simulink model "motor_modeli"  (R2024a)
settings: Solver=ode23  StartTime=0.0  StopTime=100  FixedStep=0.5  RelTol=1e-3
values from neighbouring files (symbols this model uses):
  B = 0.0001    [Motor_verileri.m]    (also in deneme1_proje_z.m)
  J = 0.004    [Motor_verileri.m]    (also in deneme1_proje_z.m = 0.0001)
  Kd = 0.000033    (= 3.3e-05)    [Motor_verileri.m]
  Ke = 0.12    [Motor_verileri.m]    (also in deneme1_proje_z.m = 0.05)
  Ki = 2.43    [Motor_verileri.m]
  Kp = 0.0114    [Motor_verileri.m]
  Kt = 0.12    [Motor_verileri.m]    (also in deneme1_proje_z.m = 0.05)
  L = 0.00005    (= 5e-05)    [Motor_verileri.m]    (also in deneme1_proje_z.m)
  R = 0.017    [Motor_verileri.m]    (also in deneme1_proje_z.m)
libraries: simulink x1
settings Model: Creator=user  LastModifiedBy=user

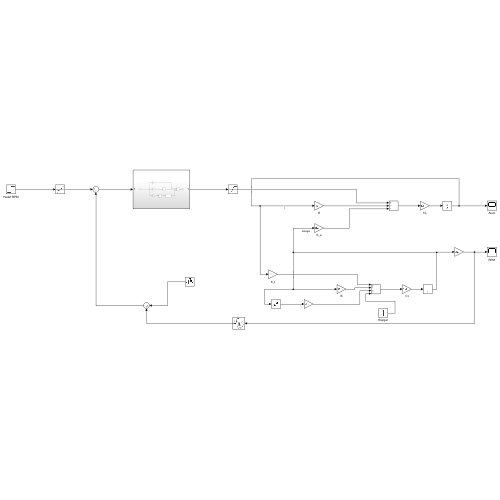
[thumbnail: Simulink's stored preview of the top-level diagram]
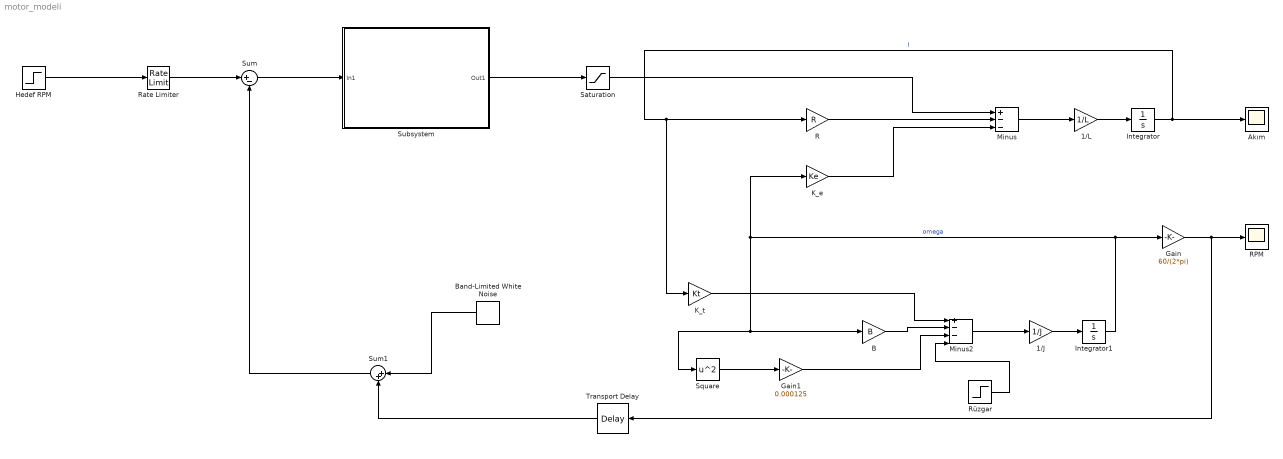
== system motor_modeli ==
  1/J : Gain  Gain=1/J
  1/L : Gain  Gain=1/L
  Akım : Scope
  B : Gain  Gain=B
  Band-Limited White Noise : simulink/Sources/Band-Limited White Noise  Cov=[0.0001]  Ts=0.1  seed=[23341]
  Gain : Gain  Gain=60/(2*pi)
  Gain1 : Gain  Gain=0.000125
  Hedef RPM : Step  Time=0.1  After=3000  SampleTime=0
  Integrator : Integrator
  Integrator1 : Integrator
  K_e : Gain  Gain=Ke
  K_t : Gain  Gain=Kt
  Minus : Sum  Inputs=+--
  Minus2 : Sum  Inputs=+---
  R : Gain  Gain=R
  RPM : Scope
  Rate Limiter : RateLimiter  RisingSlewLimit=1000  FallingSlewLimit=-1000  SampleTimeMode=inherited
  Rüzgar : Step  Time=0.5  After=5  SampleTime=0
  Saturation : Saturate  UpperLimit=60  LowerLimit=0
  Square : Math  Operator=square
  Subsystem : Subsystem
  Sum : Sum  Inputs=|+-
  Sum1 : Sum  Inputs=|++
  Transport Delay : TransportDelay  DelayTime=0.005
  wires:
  R/1 -> Minus/2
  K_e/1 -> Minus/3
  Minus/1 -> 1/L/1
  1/L/1 -> Integrator/1
  Integrator/1 -> K_t/1, R/1, Akım/1  "I"
  K_t/1 -> Minus2/1
  Minus2/1 -> 1/J/1
  Gain1/1 -> Minus2/3
  Integrator1/1 -> K_e/1, Square/1, B/1, Gain/1  "omega"
  B/1 -> Minus2/2
  1/J/1 -> Integrator1/1
  Square/1 -> Gain1/1
  Hedef RPM/1 -> Rate Limiter/1
  Sum/1 -> Subsystem/1(In1)
  Subsystem/1(Out1) -> Saturation/1
  Saturation/1 -> Minus/1
  Band-Limited White Noise/1 -> Sum1/1
  Gain/1 -> Transport Delay/1, RPM/1
  Rüzgar/1 -> Minus2/4
  Transport Delay/1 -> Sum1/2
  Rate Limiter/1 -> Sum/1
  Sum1/1 -> Sum/2

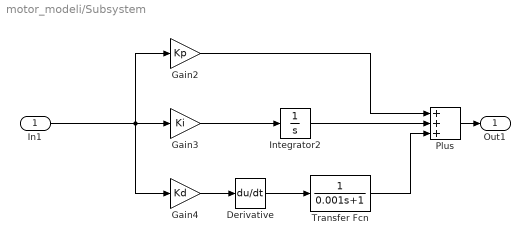
== system motor_modeli/Subsystem ==
  In1 : Inport
  Derivative : Derivative
  Gain2 : Gain  Gain=Kp
  Gain3 : Gain  Gain=Ki
  Gain4 : Gain  Gain=Kd
  Integrator2 : Integrator  LimitOutput=on  UpperSaturationLimit=60  LowerSaturationLimit=0
  Plus : Sum  Inputs=+++
  Transfer Fcn : TransferFcn  Denominator=[0.001 1]
  Out1 : Outport
  wires:
  In1/1 -> Gain2/1, Gain4/1, Gain3/1
  Gain4/1 -> Derivative/1
  Integrator2/1 -> Plus/2
  Gain2/1 -> Plus/1
  Gain3/1 -> Integrator2/1
  Plus/1 -> Out1/1
  Derivative/1 -> Transfer Fcn/1
  Transfer Fcn/1 -> Plus/3
